simulink model "Full_model_lookup_table_spring_stiffness"  (R2018a)
settings: Solver=VariableStepAuto  StartTime=0.0  StopTime=10.0  FixedStep=0.00000001  MaxStep=0.0001  RelTol=1e-3
values from neighbouring files (symbols this model uses):
  bs = 2000    [suspensiondata.mat]
  bse = 3000    [suspensiondata.mat]
  Kse = 8000    [suspensiondata.mat]
  Kt = 125000    [suspensiondata.mat]
  Ms = 250    [suspensiondata.mat]
  Mse = 90    [suspensiondata.mat]
  Mu = 40    [suspensiondata.mat]
  p1_150_p2_30v = [9.36492633169e-06 0.00052288405136 0.00126203754344 0.00219289677269 0.00306560277016 0.00370561433637 0.00457832033384 0.00562556753081 0.00667289623196 0.00766199019716 0.0087673906259 0.00987279105464 ... (306 elements, 153x2)]    [suspension_sys_data.mat]    (also in suspensiondata.mat)
  Zr = 0.2    [suspensiondata.mat]
libraries: simulink x1
settings Model: Creator=Saurabh Suman  LastModifiedBy=Saurabh Suman
settings DebuggingCC: SignalInfNanChecking=error

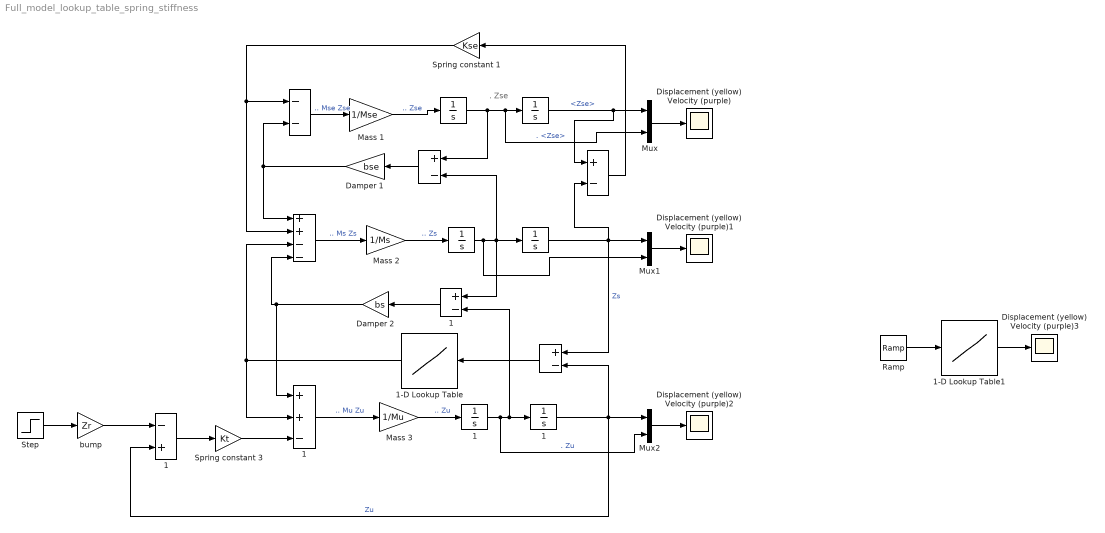
== system Full_model_lookup_table_spring_stiffness ==
  note: .
      | Zse
  " " : Integrator
  "  " : Sum  Inputs=+-
  "     " : Integrator
  "      " : Sum  Inputs=++--
  "       " : Sum  Inputs=--
  "        " : Sum  Inputs=+-
  "         " : Integrator
  "          " : Integrator
  "             " : Sum  Inputs=+-
  "             1" : Sum  Inputs=+-
  "          1" : Integrator
  "         1" : Integrator
  "       1" : Sum  Inputs=-+
  "      1" : Sum  Inputs=++-
  1-D Lookup Table : Lookup_n-D  NumberOfTableDimensions=1  LookupTableObject=p1_150_p2_30v  BreakpointsForDimension1=p1_150_p2_30v(:,1)  Table=p1_150_p2_30v(:,2)  DiagnosticForOutOfRangeInput=Warning  InternalRulePriority=Speed  RndMeth=Simplest  InputSameDT=on
  1-D Lookup Table1 : Lookup_n-D  NumberOfTableDimensions=1  LookupTableObject=p1_150_p2_30v  BreakpointsForDimension1=p1_150_p2_30v(:,1)'  Table=p1_150_p2_30v(:,2)'  InternalRulePriority=Speed  RndMeth=Simplest  InputSameDT=on
  Damper 1 : Gain  Gain=bse
  Damper 2 : Gain  Gain=bs
  Displacement (yellow) Velocity (purple){,1..3} (4 alike) : Scope
  Mass 1 : Gain  Gain=1/Mse
  Mass 2 : Gain  Gain=1/Ms
  Mass 3 : Gain  Gain=1/Mu
  Mux : Mux  Inputs=2
  Mux1 : Mux  Inputs=2
  Mux2 : Mux  Inputs=2
  Ramp : simulink/Sources/Ramp  slope=1  start=0  InitialOutput=0
  Spring constant 1 : Gain  Gain=Kse
  Spring constant 3 : Gain  Gain=Kt
  Step : Step  SampleTime=0
  bump : Gain  Gain=Zr
  wires:
  Mux1/1 -> Displacement (yellow) Velocity (purple)1/1
  Mux/1 -> Displacement (yellow) Velocity (purple)/1
  "     "/1 -> "  "/1, Mux/1  "<Zse>"
  "       1"/1 -> Spring constant 3/1
  " "/1 -> "        "/1, "     "/1, Mux/2  ". <Zse>"
  Mass 1/1 -> " "/1  ".. Zse"
  Damper 1/1 -> "      "/1, "       "/2
  Damper 2/1 -> "      "/4, "      1"/1
  Spring constant 3/1 -> "      1"/3
  "          "/1 -> Mux1/1, "  "/2, "             "/1  "Zs"
  "      1"/1 -> Mass 3/1  ".. Mu Zu"
  "       "/1 -> Mass 1/1  ".. Mse Zse"
  Mass 3/1 -> "         1"/1  ".. Zu"
  "             1"/1 -> Damper 2/1
  "  "/1 -> Spring constant 1/1
  "         1"/1 -> "          1"/1, "             1"/2, Mux2/2  ". Zu"
  Mux2/1 -> Displacement (yellow) Velocity (purple)2/1
  1-D Lookup Table/1 -> "      "/3, "      1"/2
  "          1"/1 -> "       1"/2, Mux2/1, "             "/2  "Zu"
  Spring constant 1/1 -> "      "/2, "       "/1
  "             "/1 -> 1-D Lookup Table/1
  "      "/1 -> Mass 2/1  ".. Ms Zs"
  Mass 2/1 -> "         "/1  ".. Zs"
  "         "/1 -> "        "/2, "          "/1, "             1"/1, Mux1/2
  "        "/1 -> Damper 1/1
  1-D Lookup Table1/1 -> Displacement (yellow) Velocity (purple)3/1
  Ramp/1 -> 1-D Lookup Table1/1
  bump/1 -> "       1"/1
  Step/1 -> bump/1
